simulink model "range_limiter"  (R2021b)
settings: Solver=VariableStepAuto  StartTime=0.0  StopTime=10.0  RelTol=1e-3
settings Model: Creator=mluser  LastModifiedBy=mluser

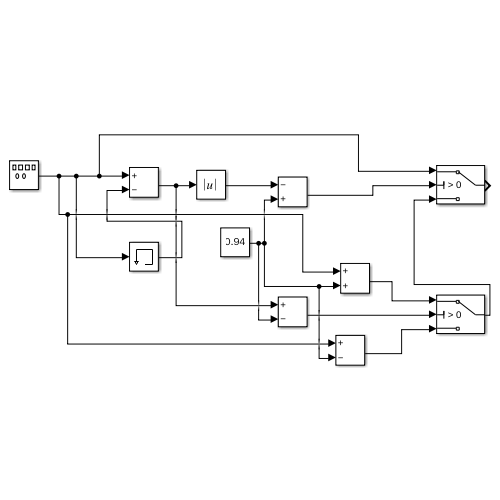
[thumbnail: Simulink's stored preview of the top-level diagram]
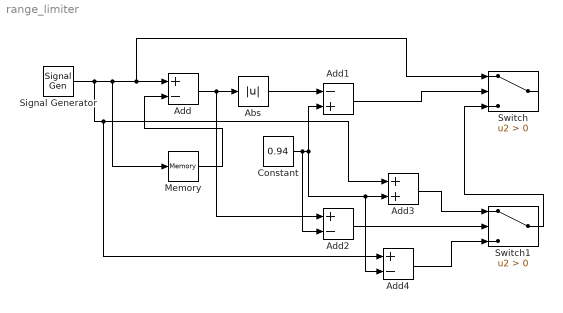
== system range_limiter ==
  Abs : Abs
  Add : Sum  Inputs=+-
  Add1 : Sum  Inputs=-+
  Add2 : Sum  Inputs=+-
  Add3 : Sum
  Add4 : Sum  Inputs=+-
  Constant : Constant  Value=0.94
  Memory : Memory
  Signal Generator : SignalGenerator  Units=rad/sec
  Switch : Switch  Criteria=u2 > Threshold
  Switch1 : Switch  Criteria=u2 > Threshold
  wires:
  Signal Generator/1 -> Add4/1, Add3/1, Memory/1, Switch/1, Add/1
  Memory/1 -> Add/2
  Abs/1 -> Add1/1
  Constant/1 -> Add2/2, Add1/2, Add4/2, Add3/2
  Add1/1 -> Switch/2
  Add/1 -> Add2/1, Abs/1
  Add2/1 -> Switch1/2
  Switch1/1 -> Switch/3
  Add3/1 -> Switch1/1
  Add4/1 -> Switch1/3
